simulink model "parallelformb"  (R2024a)
settings: Solver=VariableStepAuto  StartTime=0.0  StopTime=10.0  RelTol=1e-3
settings Model: Creator=prath  LastModifiedBy=prath

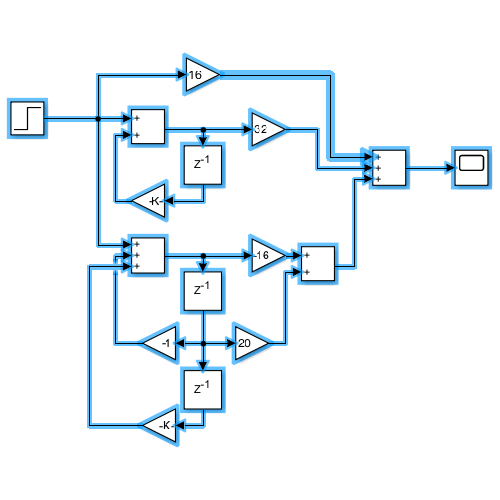
[thumbnail: Simulink's stored preview of the top-level diagram]
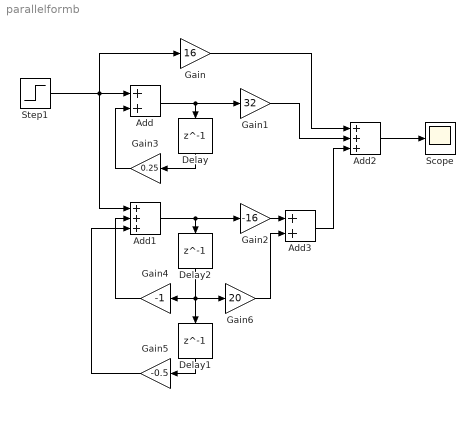
== system parallelformb ==
  Add : Sum
  Add1 : Sum  Inputs=+++
  Add2 : Sum  Inputs=+++
  Add3 : Sum
  Delay : Delay  DelayLength=1
  Delay1 : Delay  DelayLength=1
  Delay2 : Delay  DelayLength=1
  Gain : Gain  Gain=16
  Gain1 : Gain  Gain=32
  Gain2 : Gain  Gain=-16
  Gain3 : Gain  Gain=0.25
  Gain4 : Gain  Gain=-1
  Gain5 : Gain  Gain=-0.5
  Gain6 : Gain  Gain=20
  Scope : Scope
  Step1 : Step  SampleTime=0
  wires:
  Gain4/1 -> Add1/2
  Gain2/1 -> Add3/1
  Add1/1 -> Gain2/1, Delay2/1
  Delay/1 -> Gain3/1
  Gain5/1 -> Add1/3
  Add3/1 -> Add2/3
  Add/1 -> Gain1/1, Delay/1
  Step1/1 -> Add1/1, Gain/1, Add/1
  Gain1/1 -> Add2/2
  Delay1/1 -> Gain5/1
  Delay2/1 -> Gain6/1, Delay1/1, Gain4/1
  Gain3/1 -> Add/2
  Gain6/1 -> Add3/2
  Add2/1 -> Scope/1
  Gain/1 -> Add2/1
